simulink model "Tele_1DOF"  (Simulink 8.6)
settings: Solver=VariableStepAuto  StartTime=0.0  StopTime=50  FixedStep=0.005  RelTol=1e-3
values from neighbouring files (symbols this model uses):
  gamma = 0.01    [Parameters.m]
  K = ceil(max(K1,K2))    [Gains.m]
  Mm = 1.4571    [Parameters.m]
  Ms = 2.9142    [Parameters.m]
  P = 10    [Parameters.m]
undefined symbols (not defined in the file or in its folder): dm, ds, pm0, ps0, threshold, vm0, vs0
settings Model: Creator=TOSHIBA  LastModifiedBy=TOSHIBA
settings DataIOCC: SaveFormat=Dataset  SignalLoggingSaveFormat=Dataset
settings OptimizationCC: ExpressionDepthLimit=128
settings DebuggingCC: UnderspecifiedInitializationDetection=Simplified  MergeDetectMultiDrivingBlocksExec=error  SolverPrmCheckMsg=none  FcnCallInpInsideContextMsg=EnableAllAsError  StateNameClashWarn=none
settings HardwareCC: ProdBitPerPointer=64  ProdLargestAtomicFloat=Float  ProdIntDivRoundTo=Zero  ProdEndianess=LittleEndian  ProdWordSize=64  ProdHWDeviceType=Intel->x86-64 (Windows64)
settings GRTTargetCC: GeneratePreprocessorConditionals=Use local settings  CombineOutputUpdateFcns=on  GRTInterface=off
settings ConfigComp: CovModelRefEnable=off

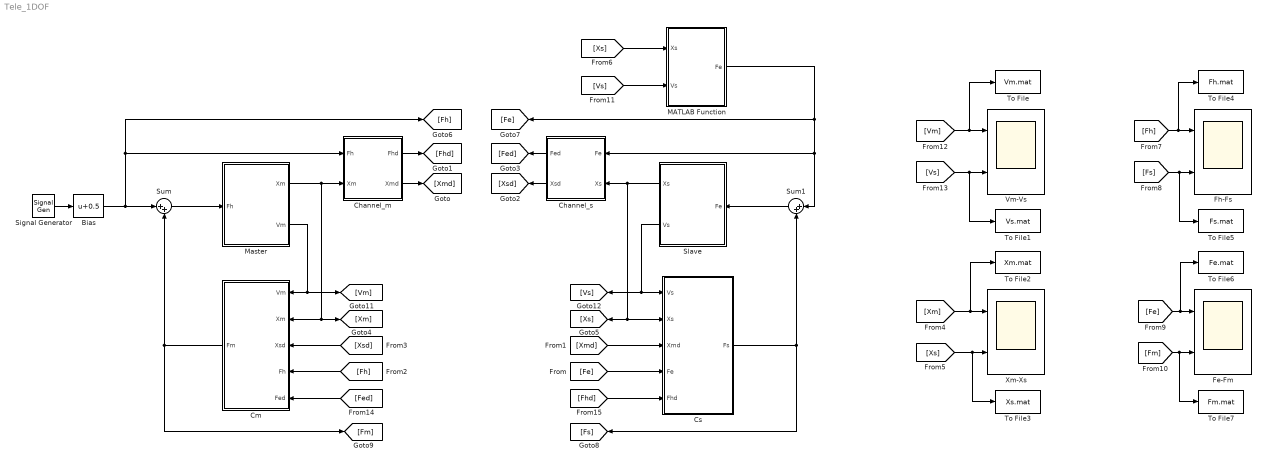
== system Tele_1DOF ==
  Bias : Bias  Bias=0.5
  Channel_m : Subsystem
  Channel_s : Subsystem
  Cm : Subsystem
  Cs : Subsystem
  Fe-Fm : Scope  NumInputPorts=2
  Fh-Fs : Scope  NumInputPorts=2
  MATLAB Function : MATLAB Function  TreatAsAtomicUnit=on
  Master : Subsystem
  Signal Generator : SignalGenerator  Frequency=pi/10  Units=rad/sec
  Slave : Subsystem
  Sum : Sum  Inputs=|++
  Sum1 : Sum  Inputs=|++
  To File : ToFile  Filename=Vm.mat  MatrixName=Vm  SaveFormat=Timeseries
  To File1 : ToFile  Filename=Vs.mat  MatrixName=Vs  SaveFormat=Timeseries
  To File2 : ToFile  Filename=Xm.mat  MatrixName=Xm  SaveFormat=Timeseries
  To File3 : ToFile  Filename=Xs.mat  MatrixName=Xs  SaveFormat=Timeseries
  To File4 : ToFile  Filename=Fh.mat  MatrixName=Fh  SaveFormat=Timeseries
  To File5 : ToFile  Filename=Fs.mat  MatrixName=Fs  SaveFormat=Timeseries
  To File6 : ToFile  Filename=Fe.mat  MatrixName=Fe  SaveFormat=Timeseries
  To File7 : ToFile  Filename=Fm.mat  MatrixName=Fm  SaveFormat=Timeseries
  Vm-Vs : Scope  NumInputPorts=2
  Xm-Xs : Scope  NumInputPorts=2
  wires:
  Sum/1 -> Master/1(Fh)
  Signal Generator/1 -> Bias/1
  Cm/1(Fm) -> Sum/2, [Fm]
  Cs/1(Fs) -> Sum1/2, [Fs]
  Sum1/1 -> Slave/1(Fe)
  Master/1(Xm) -> [Xm], Cm/2(Xm), Channel_m/2(Xm)
  Master/2(Vm) -> [Vm], Cm/1(Vm)
  Channel_m/2(Xmd) -> [Xmd]
  Channel_m/1(Fhd) -> [Fhd]
  Channel_s/1(Fed) -> [Fed]
  Channel_s/2(Xsd) -> [Xsd]
  Slave/1(Xs) -> [Xs], Cs/2(Xs), Channel_s/2(Xs)
  Slave/2(Vs) -> [Vs], Cs/1(Vs)
  [Fe] -> Cs/4(Fe)
  [Xmd] -> Cs/3(Xmd)
  [Xsd] -> Cm/3(Xsd)
  MATLAB Function/1(Fe) -> Sum1/1, Channel_s/1(Fe), [Fe]
  Bias/1 -> Channel_m/1(Fh), [Fh], Sum/1
  [Xm] -> To File2/1, Xm-Xs/1
  [Xs] -> To File3/1, Xm-Xs/2
  [Fh] -> To File4/1, Fh-Fs/1
  [Fs] -> To File5/1, Fh-Fs/2
  [Fe] -> To File6/1, Fe-Fm/1
  [Fm] -> Fe-Fm/2, To File7/1
  [Xs] -> MATLAB Function/1(Xs)
  [Vs] -> MATLAB Function/2(Vs)
  [Vm] -> To File/1, Vm-Vs/1
  [Vs] -> To File1/1, Vm-Vs/2
  [Fhd] -> Cs/5(Fhd)
  [Fed] -> Cm/5(Fed)
  [Fh] -> Cm/4(Fh)

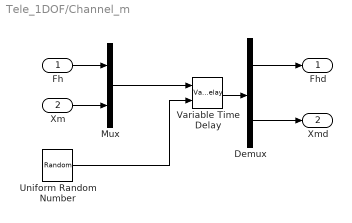
== system Tele_1DOF/Channel_m ==
  Fh : Inport
  Xm : Inport  Port=2
  Demux : Demux  Outputs=2
  Mux : Mux  Inputs=2
  Uniform Random Number : UniformRandomNumber  Minimum=0  Maximum=dm  SampleTime=0.0001
  Variable Time Delay : VariableTransportDelay  MaximumDelay=dm
  Fhd : Outport
  Xmd : Outport  Port=2
  wires:
  Uniform Random Number/1 -> Variable Time Delay/2
  Mux/1 -> Variable Time Delay/1
  Fh/1 -> Mux/1
  Demux/2 -> Xmd/1
  Demux/1 -> Fhd/1
  Variable Time Delay/1 -> Demux/1
  Xm/1 -> Mux/2

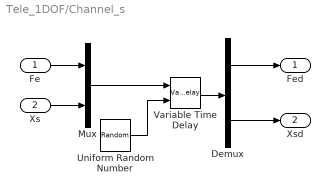
== system Tele_1DOF/Channel_s ==
  Fe : Inport
  Xs : Inport  Port=2
  Demux : Demux  Outputs=2
  Mux : Mux  Inputs=2
  Uniform Random Number : UniformRandomNumber  Minimum=0  Maximum=ds  SampleTime=0
  Variable Time Delay : VariableTransportDelay  MaximumDelay=ds
  Fed : Outport
  Xsd : Outport  Port=2
  wires:
  Xs/1 -> Mux/2
  Variable Time Delay/1 -> Demux/1
  Demux/1 -> Fed/1
  Demux/2 -> Xsd/1
  Fe/1 -> Mux/1
  Mux/1 -> Variable Time Delay/1
  Uniform Random Number/1 -> Variable Time Delay/2

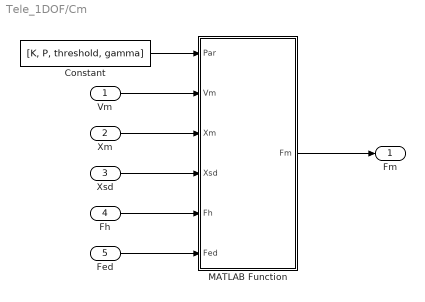
== system Tele_1DOF/Cm ==
  Vm : Inport
  Xm : Inport  Port=2
  Xsd : Inport  Port=3
  Fh : Inport  Port=4
  Fed : Inport  Port=5
  Constant : Constant  Value=[K, P, threshold, gamma]
  MATLAB Function : MATLAB Function  TreatAsAtomicUnit=on
  Fm : Outport
  wires:
  MATLAB Function/1(Fm) -> Fm/1
  Constant/1 -> MATLAB Function/1(Par)
  Xsd/1 -> MATLAB Function/4(Xsd)
  Vm/1 -> MATLAB Function/2(Vm)
  Xm/1 -> MATLAB Function/3(Xm)
  Fh/1 -> MATLAB Function/5(Fh)
  Fed/1 -> MATLAB Function/6(Fed)

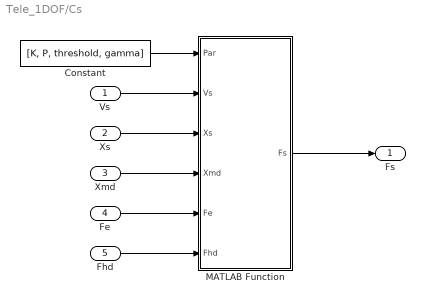
== system Tele_1DOF/Cs ==
  Vs : Inport
  Xs : Inport  Port=2
  Xmd : Inport  Port=3
  Fe : Inport  Port=4
  Fhd : Inport  Port=5
  Constant : Constant  Value=[K, P, threshold, gamma]
  MATLAB Function : MATLAB Function  TreatAsAtomicUnit=on
  Fs : Outport
  wires:
  Xs/1 -> MATLAB Function/3(Xs)
  Vs/1 -> MATLAB Function/2(Vs)
  Xmd/1 -> MATLAB Function/4(Xmd)
  Constant/1 -> MATLAB Function/1(Par)
  MATLAB Function/1(Fs) -> Fs/1
  Fe/1 -> MATLAB Function/5(Fe)
  Fhd/1 -> MATLAB Function/6(Fhd)

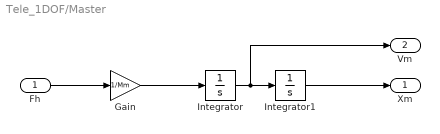
== system Tele_1DOF/Master ==
  Fh : Inport
  Gain : Gain  Gain=1/Mm
  Integrator : Integrator  InitialCondition=vm0
  Integrator1 : Integrator  InitialCondition=pm0
  Xm : Outport
  Vm : Outport  Port=2
  wires:
  Integrator/1 -> Vm/1, Integrator1/1
  Gain/1 -> Integrator/1
  Integrator1/1 -> Xm/1
  Fh/1 -> Gain/1

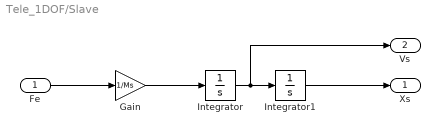
== system Tele_1DOF/Slave ==
  Fe : Inport
  Gain : Gain  Gain=1/Ms
  Integrator : Integrator  InitialCondition=vs0
  Integrator1 : Integrator  InitialCondition=ps0
  Xs : Outport
  Vs : Outport  Port=2
  wires:
  Fe/1 -> Gain/1
  Integrator1/1 -> Xs/1
  Gain/1 -> Integrator/1
  Integrator/1 -> Integrator1/1, Vs/1

== matlab function Cs/MATLAB Function ==
  data: Par input double; Fs output double; Vs input double; Xs input double; Xmd input double; Fe input double; Fhd input double
function Fs = fcn(Par,Vs, Xs, Xmd, Fe, Fhd)
%#codegen
K=Par(1);
P=Par(2);
threshold=Par(3);
gamma=Par(4);
Fs = -(P+Upsilon(threshold,gamma,Xs-Xmd,Fe+Fhd))*(Xs-Xmd)-K*Vs+Fhd;

== matlab function Cm/MATLAB Function ==
  data: Par input double; Fm output double; Vm input double; Xm input double; Xsd input double; Fh input double; Fed input double
function Fm = fcn(Par,Vm, Xm, Xsd, Fh, Fed)
%#codegen
K=Par(1);
P=Par(2);
threshold=Par(3);
gamma=Par(4);
Fm = -(P+Upsilon(threshold,gamma,Xm-Xsd,Fh+Fed))*(Xm-Xsd)-K*Vm+Fed;

== matlab function MATLAB Function ==
  data: Xs input double; Fe output double; Vs input double
function Fe = Env(Xs,Vs)
%#codegen
Pwall=0.5;
Kwall=1000;
Bwall=10;

if Xs>=Pwall
    Fe=-Kwall*(Xs-Pwall)-Bwall*Vs;
    if Fe>0
        Fe=0;
    end
else
    Fe=0;
end
